simulink model "ctrl_PF_ad"  (R2023a)
settings: Solver=FixedStepAuto  StartTime=0.0  StopTime=Tf  FixedStep=0.05  RelTol=1e-3
StopFcn:
  | save('testdata')
undefined symbols (not defined in the file or in its folder): adap, Ba_0, Bb, Bv_0, Bx_0, Cp, Cp_prime, Cpv, d, dA_BP1, dA_BP2, dA_Hull, dA_PH, dA_Sail, dA_SProot, dA_X1a, dA_X1b, dA_X2a, dA_X2b, dA_X3a, dA_X3b, dA_X4a, dA_X4b, Ixx, Ixy, Ixz, Iyy, Iyz, Izz, Ky, L1, Mb, n_BP1, n_BP2, n_Hull, n_PH, n_Sail, n_SProot, n_X2a, n_X2b, n_X3a, n_X4a, n_X4b, nt_BP1, nt_BP2, nt_Hull, nt_PH, nt_Sail, nt_SProot, nt_X1a, nt_X1b, nt_X2a, nt_X2b, nt_X3a, nt_X3b, nt_X4a, nt_X4b, Seastate, Tf, Ts ... (+50)
libraries: simulink x8, sharedtransform x2, dspmathops x2
(part 2 of 5)

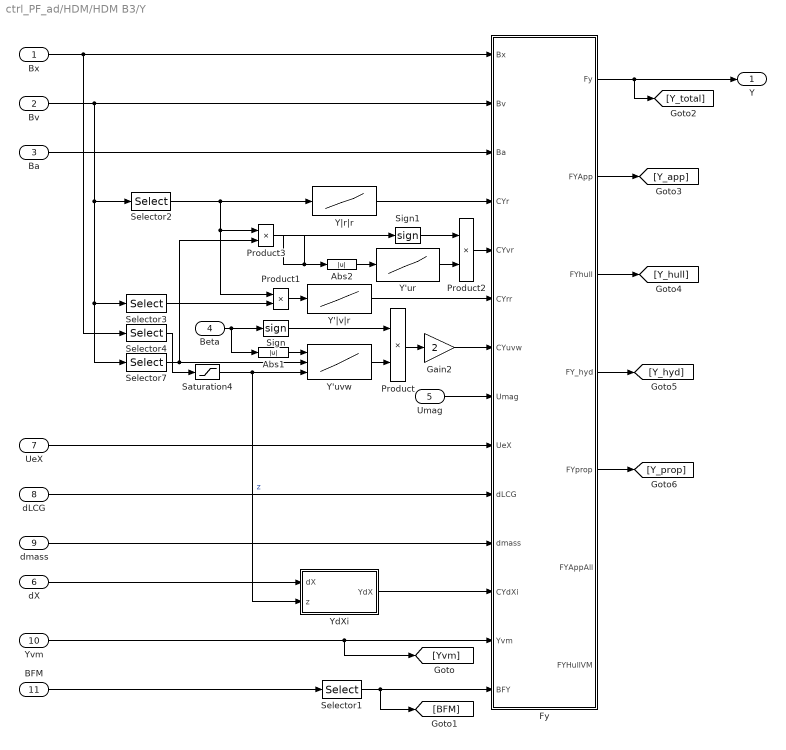
== system ctrl_PF_ad/HDM/HDM B3/Y ==
  Bx : Inport
  Bv : Inport  Port=2
  Ba : Inport  Port=3
  Beta : Inport  Port=4
  Umag : Inport  Port=5
  dX : Inport  Port=6
  UeX : Inport  Port=7
  dLCG : Inport  Port=8
  dmass : Inport  Port=9
  Yvm : Inport  Port=10
  BFM : Inport  Port=11
  Abs1 : Abs  SaturateOnIntegerOverflow=off
  Abs2 : Abs  SaturateOnIntegerOverflow=off
  Fy : MATLAB Function  TreatAsAtomicUnit=on
  Gain2 : Gain  Gain=2
  Product{,1..3} (4 alike) : Product
  Saturation4 : Saturate  UpperLimit=-13.8724  LowerLimit=-35.0624
  Selector1 : Selector  InputPortWidth=6  IndexOptions=Index vector (dialog)  Indices=2  OutputSizes=1
  Selector2 : Selector  InputPortWidth=6  IndexOptions=Index vector (dialog)  Indices=6  OutputSizes=1
  Selector3 : Selector  InputPortWidth=6  IndexOptions=Index vector (dialog)  Indices=2  OutputSizes=1
  Selector4 : Selector  InputPortWidth=6  IndexOptions=Index vector (dialog)  Indices=3  OutputSizes=1
  Selector7 : Selector  InputPortWidth=6  IndexOptions=Index vector (dialog)  Indices=1  OutputSizes=1
  Sign : Signum
  Sign1 : Signum
  Y'ur : Lookup_n-D  NumberOfTableDimensions=1  BreakpointsForDimension1=|  Table=|  InternalRulePriority=Speed  RndMeth=Simplest
      BreakpointsForDimension1=|
      | [0.03999989
      | 0.079999993
      | 0.11999963
      | 0.15999956]
      Table=|
      | [-5.2094E-04
      | -1.0594E-03
      | -1.5649E-03
      | -2.0981E-03]
  Y'uvw : Lookup_n-D  NumberOfTableDimensions=3  BreakpointsForDimension1=|  BreakpointsForDimension2=|  BreakpointsForDimension3=|  Table=|  InternalRulePriority=Speed  RndMeth=Simplest
      BreakpointsForDimension1=|
      | [0
      | 4
      | 8
      | 12]
      BreakpointsForDimension2=|
      | [-5.1444E+00
      | -3.0866E+00
      | -1.5433E+00
      | ]
      Table=|
      | reshape([0.0000000E+00
      | -5.0280621E-03
      | -9.4175348E-03
      | -1.4397458E-02
      | 0.0000000E+00
      | -5.0037454E-03
      | -9.1645405E-03
      | -1.4507402E-02
      | 0.0000000E+00
      | -4.2819107E-03
      | -9.0361786E-03
      | -1.4507235E-02
      | 0.0000000E+00
      | -4.7723270E-03
      | -9.7378407E-03
      | -1.5377541E-02
      | 0.0000000E+00
      | -4.7276301E-03
      | -9.6949815E-03
      | -1.5393721E-02
      | 0.0000000E+00
      | -4.5359209E-03
      | -9.4966039E-03
      | -1.6947859E-02
      | 0.0000000E+00
      | -5.1295007E-03
      | -1.0575377E-02
      | -1.6672924E-02
      | 0.0000000E+00
      | -4.9811404E-03
      | -1.0209461E-02
      | -1.6298327E-02
      | 0.0000000E+00
      | -4.7780219E-03
      | -1.0008968E-02
      | -1.6115181E-02
      | 0.0000000E+00
      | -5.7252015E-03
      | -1.1973447E-02
      | -1.9152812E-02
      | 0.0000000E+00
      | -5.2128737E-03
      | -1.0845978E-02
      | -1.7281669E-02
      | 0.0000000E+00
      | -4.9979037E-03
      | -1.0845685E-02
      | -1.6944141E-02],[4,3,4])
      BreakpointsForDimension3=|
      | [-35.0624 -18.3724 -15.3724 -13.8724
      | ]
      settings: InputPortMap=u0,u1,u2
  Y'|v|r : Lookup_n-D  NumberOfTableDimensions=1  BreakpointsForDimension1=|  Table=|  InternalRulePriority=Speed  RndMeth=Simplest
      BreakpointsForDimension1=|
      | [-0.0015
      | -0.0012
      | -0.0009
      | -0.0006
      | -0.0003
      | -0.0001
      | 0.0001
      | 0.0003
      | 0.0006
      | 0.0009
      | 0.0012
      | 0.0015]
      Table=|
      | [-2.9784E-01
      | -2.6725E-01
      | -2.3292E-01
      | -2.0077E-01
      | -1.1489E-01
      | -7.6673E-03
      | -7.5516E-03
      | -1.1617E-01
      | -2.0077E-01
      | -2.9128E-01
      | -3.5974E-01
      | -4.7839E-01]
  YdXi : Subsystem
  Y|r|r : Lookup_n-D  NumberOfTableDimensions=1  BreakpointsForDimension1=|  Table=|  InternalRulePriority=Speed  RndMeth=Simplest
      BreakpointsForDimension1=|
      | [-0.02
      | -0.015
      | -0.012958963
      | -0.009719222
      | -0.006479482
      | -0.003239741
      | -0.00161987
      | -0.000647948
      | 0.000647948
      | 0.00161987
      | 0.003239741
      | 0.006479482
      | 0.009719222
      | 0.012958963
      | 0.015
      | 0.02
      | ]
      Table=|
      | [3.6478E-03
      | 3.8686E-03
      | 3.4313E-03
      | 4.0790E-03
      | 3.9500E-03
      | 3.6018E-03
      | 3.6796E-03
      | 3.5502E-03
      | 3.4310E-03
      | 3.4872E-03
      | 4.2239E-03
      | 4.0934E-03
      | 3.0314E-03
      | 2.5726E-03
      | 2.9188E-03
      | 2.7740E-03
      | ]
  Y : Outport
  wires:
  Fy/5(FYprop) -> [Y_prop]
  Fy/4(FY_hyd) -> [Y_hyd]
  Fy/3(FYhull) -> [Y_hull]
  Fy/2(FYApp) -> [Y_app]
  YdXi/1(YdX) -> Fy/12(CYdXi)
  Saturation4/1 -> Y'uvw/3, YdXi/2(z)  "z"
  Selector1/1 -> Fy/14(BFY), [BFM]
  BFM/1 -> Selector1/1
  Yvm/1 -> [Yvm], Fy/13(Yvm)
  Gain2/1 -> Fy/7(CYuvw)
  Product/1 -> Gain2/1
  Abs2/1 -> Y'ur/1
  Sign1/1 -> Product2/1
  Product2/1 -> Fy/5(CYvr)
  Abs1/1 -> Y'uvw/1
  Sign/1 -> Product/1
  Y'uvw/1 -> Product/2
  Selector4/1 -> Saturation4/1
  Y'ur/1 -> Product2/2
  Y|r|r/1 -> Fy/4(CYr)
  Fy/1(Fy) -> Y/1, [Y_total]
  Y'|v|r/1 -> Fy/6(CYrr)
  Selector2/1 -> Y|r|r/1, Product3/1, Product1/1
  Product1/1 -> Y'|v|r/1
  Product3/1 -> Abs2/1, Sign1/1
  dX/1 -> YdXi/1(dX)
  dmass/1 -> Fy/11(dmass)
  dLCG/1 -> Fy/10(dLCG)
  Ba/1 -> Fy/3(Ba)
  Selector3/1 -> Product1/2
  UeX/1 -> Fy/9(UeX)
  Bx/1 -> Selector4/1, Fy/1(Bx)
  Umag/1 -> Fy/8(Umag)
  Bv/1 -> Selector7/1, Selector3/1, Selector2/1, Fy/2(Bv)
  Beta/1 -> Abs1/1, Sign/1
  Selector7/1 -> Product3/2, Y'uvw/2

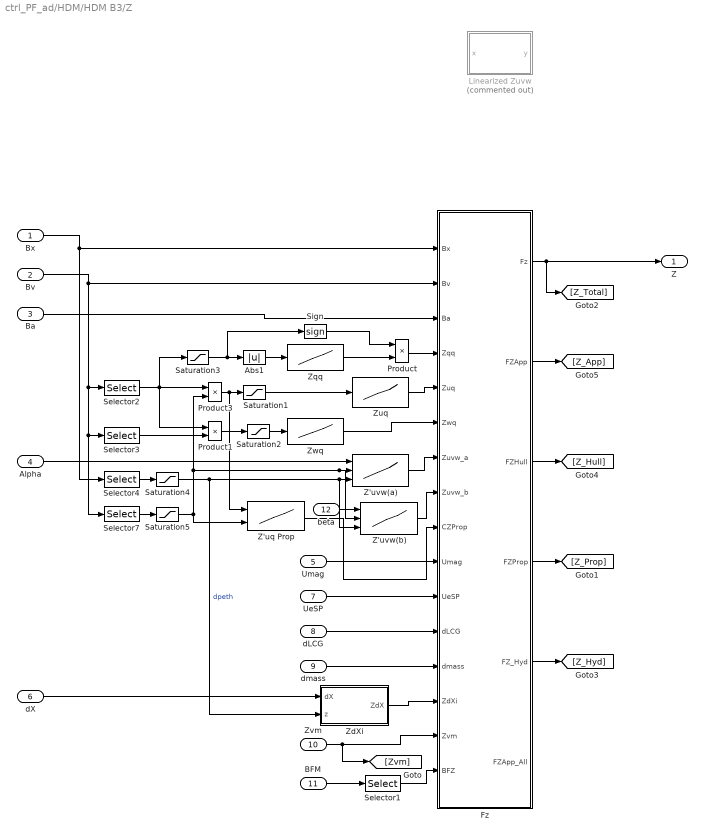
== system ctrl_PF_ad/HDM/HDM B3/Z ==
  Bx : Inport
  Bv : Inport  Port=2
  Ba : Inport  Port=3
  Alpha : Inport  Port=4
  Umag : Inport  Port=5
  dX : Inport  Port=6
  UeSP : Inport  Port=7
  dLCG : Inport  Port=8
  dmass : Inport  Port=9
  Zvm : Inport  Port=10
  BFM : Inport  Port=11
  beta : Inport  Port=12
  Abs1 : Abs  SaturateOnIntegerOverflow=off
  Fz : MATLAB Function  TreatAsAtomicUnit=on
  Linearized Zuvw : MATLAB Function  Commented=on  TreatAsAtomicUnit=on
  Product : Product
  Product1 : Product
  Product3 : Product
  Saturation1 : Saturate  UpperLimit=0.04  LowerLimit=-0.04
  Saturation2 : Saturate  UpperLimit=0.0015  LowerLimit=-0.0015
  Saturation3 : Saturate  UpperLimit=0.02  LowerLimit=-0.02
  Saturation4 : Saturate  UpperLimit=-13.8724  LowerLimit=-35.0624
  Saturation5 : Saturate  UpperLimit=-1.5433E+00  LowerLimit=-5.14444
  Selector1 : Selector  InputPortWidth=6  IndexOptions=Index vector (dialog)  Indices=3  OutputSizes=1
  Selector2 : Selector  InputPortWidth=6  IndexOptions=Index vector (dialog)  Indices=5  OutputSizes=1
  Selector3 : Selector  InputPortWidth=6  IndexOptions=Index vector (dialog)  Indices=3  OutputSizes=1
  Selector4 : Selector  InputPortWidth=6  IndexOptions=Index vector (dialog)  Indices=3  OutputSizes=1
  Selector7 : Selector  InputPortWidth=6  IndexOptions=Index vector (dialog)  Indices=1  OutputSizes=1
  Sign : Signum
  Z'uq Prop : Lookup_n-D  BreakpointsForDimension1=|  BreakpointsForDimension2=[-7.71666 -5.14444 -3.086664 -1.543332]  Table=|  InternalRulePriority=Speed  RndMeth=Simplest
      BreakpointsForDimension1=|
      | [-2.0E-01
      | -1.5E-01
      | -1.0E-01
      | -5.0E-02
      | 0.0E+00
      | 5.0E-02
      | 1.0E-01
      | 1.5E-01
      | 2.0E-01
      | ]
      Table=|
      | reshape([1.3913E-04
      | 1.0452E-04
      | 6.9900E-05
      | 3.5283E-05
      | 6.6700E-07
      | -3.3949E-05
      | -6.8566E-05
      | -1.0318E-04
      | -1.3780E-04
      | 2.8914E-04
      | 2.1702E-04
      | 1.4490E-04
      | 7.2785E-05
      | 6.6700E-07
      | -7.1451E-05
      | -1.4357E-04
      | -2.1569E-04
      | -2.8780E-04
      | 1.1606E-04
      | 8.7208E-05
      | 5.8361E-05
      | 2.9514E-05
      | 6.6700E-07
      | -2.8180E-05
      | -5.7027E-05
      | -8.5874E-05
      | -1.1472E-04
      | 1.1606E-04
      | 8.7208E-05
      | 5.8361E-05
      | 2.9514E-05
      | 6.6700E-07
      | -2.8180E-05
      | -5.7027E-05
      | -8.5874E-05
      | -1.1472E-04],[9,4])
      settings: InputPortMap=u0,u1
  Z'uvw(a) : Lookup_n-D  NumberOfTableDimensions=3  BreakpointsForDimension1=|  BreakpointsForDimension2=|  BreakpointsForDimension3=|  Table=|  InternalRulePriority=Speed  RndMeth=Simplest
      BreakpointsForDimension1=|
      | [-12
      | -8
      | -4
      | 0
      | 4
      | 8
      | 12]
      BreakpointsForDimension2=|
      | [-5.1444E+00
      | -3.0866E+00
      | -1.5433E+00
      | ]
      Table=|
      | reshape([-3.82587E-03
      | -2.42543E-03
      | -1.05453E-03
      | 1.94202E-04
      | 1.48991E-03
      | 3.04047E-03
      | 4.14104E-03
      | -3.76348E-03
      | -2.38508E-03
      | -9.82619E-04
      | 1.94202E-04
      | 1.47560E-03
      | 3.02863E-03
      | 4.06663E-03
      | -3.75964E-03
      | -2.29001E-03
      | -8.34074E-04
      | 1.94202E-04
      | 1.38956E-03
      | 2.91153E-03
      | 4.15251E-03
      | -3.11218E-03
      | -1.80502E-03
      | -4.97855E-04
      | 8.09305E-04
      | 2.11647E-03
      | 3.42363E-03
      | 4.73079E-03
      | -2.62573E-03
      | -1.48072E-03
      | -3.35708E-04
      | 8.09305E-04
      | 1.95432E-03
      | 3.09933E-03
      | 4.24434E-03
      | -2.06413E-03
      | -1.10632E-03
      | -1.48507E-04
      | 8.09305E-04
      | 1.76712E-03
      | 2.72493E-03
      | 3.68274E-03
      | -3.09997E-03
      | -1.76300E-03
      | -4.26025E-04
      | 9.10947E-04
      | 2.24792E-03
      | 3.58489E-03
      | 4.92186E-03
      | -2.49055E-03
      | -1.35672E-03
      | -2.22886E-04
      | 9.10947E-04
      | 2.04478E-03
      | 3.17861E-03
      | 4.31245E-03
      | -2.64104E-03
      | -1.45704E-03
      | -2.73048E-04
      | 9.10947E-04
      | 2.09494E-03
      | 3.27894E-03
      | 4.46293E-03
      | -0.003059752
      | -0.001711935
      | -0.000364117
      | 0.0009837
      | 0.002331518
      | 0.003679335
      | 0.005027153
      | -0.002351082
      | -0.0012256
      | -0.000100118
      | 0.0009837
      | 0.002109182
      | 0.003234664
      | 0.004360146
      | -0.001725739
      | -0.000822593
      | 8.05539E-05
      | 0.0009837
      | 0.001886847
      | 0.002789993
      | 0.00369314],[7,3,4])
      BreakpointsForDimension3=|
      | [-35.0624 -18.3724 -15.3724 -13.8724
      | ]
      settings: InputPortMap=u0,u1,u2
  Z'uvw(b) : Lookup_n-D  NumberOfTableDimensions=3  BreakpointsForDimension1=|  BreakpointsForDimension2=|  BreakpointsForDimension3=|  Table=|  InternalRulePriority=Speed  RndMeth=Simplest
      BreakpointsForDimension1=|
      | [0
      | 4
      | 8
      | 12]
      BreakpointsForDimension2=|
      | [-5.1444E+00
      | -3.0866E+00
      | -1.5433E+00
      | ]
      Table=|
      | reshape([0.0000000E+00
      | -5.9986916E-04
      | -2.7503348E-03
      | -5.0777589E-03
      | 0.0000000E+00
      | -6.0654884E-04
      | -2.4512564E-03
      | -5.2464901E-03
      | 0.0000000E+00
      | -7.6137528E-04
      | -2.4084463E-03
      | -5.2118678E-03
      | 0.0000000E+00
      | -8.2427914E-04
      | -2.5250249E-03
      | -5.3103563E-03
      | 0.0000000E+00
      | -8.1036019E-04
      | -2.5315266E-03
      | -5.5141459E-03
      | 0.0000000E+00
      | -7.9799041E-04
      | -2.5595242E-03
      | -5.2319004E-03
      | 0.0000000E+00
      | -8.6989011E-04
      | -2.5865820E-03
      | -5.6151595E-03
      | 0.0000000E+00
      | -8.4361582E-04
      | -2.6124115E-03
      | -5.7143353E-03
      | 0.0000000E+00
      | -8.2567611E-04
      | -2.6088331E-03
      | -5.6150660E-03
      | 0.0000000E+00
      | -9.1003224E-04
      | -2.7683191E-03
      | -6.0189061E-03
      | 0.0000000E+00
      | -8.4211433E-04
      | -2.5899187E-03
      | -5.7497784E-03
      | 0.0000000E+00
      | -8.2014014E-04
      | -2.4092466E-03
      | -5.6643347E-03],[4,3,4])
      BreakpointsForDimension3=|
      | [-35.0624 -18.3724 -15.3724 -13.8724
      | ]
      settings: InputPortMap=u0,u1,u2
  ZdXi : Subsystem
  Zqq : Lookup_n-D  NumberOfTableDimensions=1  BreakpointsForDimension1=|  Table=|  InternalRulePriority=Speed  RndMeth=Simplest
      BreakpointsForDimension1=|
      | [0.000127901
      | 0.000383704
      | 0.000639507
      | 0.001279013
      | 0.002558026
      | ]
      Table=|
      | [-1.5611E-03
      | -1.0379E-04
      | 3.9238E-05
      | 1.1475E-04
      | 1.3579E-04
      | ]
  Zuq : Lookup_n-D  NumberOfTableDimensions=1  BreakpointsForDimension1=|  Table=|  InternalRulePriority=Speed  RndMeth=Simplest
      BreakpointsForDimension1=|
      | [-0.04
      | -0.03
      | -0.02
      | -0.01
      | -0.005
      | -0.002
      | 0.002
      | 0.005
      | 0.01
      | 0.02
      | 0.03
      | 0.04
      | ]
      Table=|
      | [-9.8908E-03
      | -9.0784E-03
      | -8.9566E-03
      | -1.0733E-02
      | -1.4141E-02
      | -2.4189E-02
      | -6.5605E-03
      | -7.1594E-03
      | -7.6366E-03
      | -7.9008E-03
      | -6.1794E-03
      | -6.1029E-03
      | ]
  Zwq : Lookup_n-D  NumberOfTableDimensions=1  BreakpointsForDimension1=|  Table=|  InternalRulePriority=Speed  RndMeth=Simplest
      BreakpointsForDimension1=|
      | [-0.0015
      | -0.0012
      | -0.0009
      | -0.0006
      | -0.0003
      | -0.0001
      | 0.0001
      | 0.0003
      | 0.0006
      | 0.0009
      | 0.0012
      | 0.0015]
      Table=|
      | [-2.9784E-01
      | -2.6725E-01
      | -2.3292E-01
      | -2.0077E-01
      | -1.1489E-01
      | -7.6673E-03
      | -7.5516E-03
      | -1.1617E-01
      | -2.0077E-01
      | -2.9128E-01
      | -3.5974E-01
      | -4.7839E-01]
  Z : Outport
  wires:
  beta/1 -> Z'uvw(b)/1
  Z'uvw(b)/1 -> Fz/8(Zuvw_b)
  Product/1 -> Fz/4(Zqq)
  Sign/1 -> Product/1
  Abs1/1 -> Zqq/1
  Selector7/1 -> Saturation5/1
  Saturation5/1 -> Z'uq Prop/2, Z'uvw(b)/2, Z'uvw(a)/2, Product3/2
  Saturation4/1 -> ZdXi/2(z), Z'uvw(a)/3, Z'uvw(b)/3  "dpeth"
  Fz/5(FZ_Hyd) -> [Z_Hyd]
  Fz/4(FZProp) -> [Z_Prop]
  Fz/3(FZHull) -> [Z_Hull]
  Fz/2(FZApp) -> [Z_App]
  ZdXi/1(ZdX) -> Fz/14(ZdXi)
  Selector1/1 -> Fz/16(BFZ)
  BFM/1 -> Selector1/1
  Z'uvw(a)/1 -> Fz/7(Zuvw_a)
  Zqq/1 -> Product/2
  Z'uq Prop/1 -> Fz/9(CZProp)
  Zwq/1 -> Fz/6(Zwq)
  Selector2/1 -> Saturation3/1, Product1/1, Product3/1
  Alpha/1 -> Z'uvw(a)/1
  Bv/1 -> Selector7/1, Selector3/1, Selector2/1, Fz/2(Bv)
  Umag/1 -> Fz/10(Umag)
  Bx/1 -> Selector4/1, Fz/1(Bx)
  Product3/1 -> Z'uq Prop/1, Saturation1/1
  UeSP/1 -> Fz/11(UeSP)
  Selector3/1 -> Product1/2
  Product1/1 -> Saturation2/1
  dLCG/1 -> Fz/12(dLCG)
  dmass/1 -> Fz/13(dmass)
  dX/1 -> ZdXi/1(dX)
  Saturation1/1 -> Zuq/1
  Saturation2/1 -> Zwq/1
  Saturation3/1 -> Sign/1, Abs1/1
  Fz/1(Fz) -> [Z_Total], Z/1
  Zuq/1 -> Fz/5(Zuq)
  Ba/1 -> Fz/3(Ba)
  Zvm/1 -> [Zvm], Fz/15(Zvm)
  Selector4/1 -> Saturation4/1

== system ctrl_PF_ad/HDM/Integration and Coord. Transfrom/Coordinate Transform ==
  Bv : Inport
  Integrator : Integrator  InitialCondition=Bx_0
  MATLAB Function2 : MATLAB Function  TreatAsAtomicUnit=on
  X_earth : Outport  VectorParamsAs1DForOutWhenUnconnected=off
  wires:
  MATLAB Function2/1(out) -> Integrator/1
  Bv/1 -> MATLAB Function2/2(Bv)
  Integrator/1 -> X_earth/1, MATLAB Function2/1(Bx)

== system ctrl_PF_ad/HDM/Integration and Coord. Transfrom/Rigid Body Motion ==
  F_hyd : Inport
  Bx : Inport  Port=2
  Demux : Demux  Outputs=6
  Demux1 : Demux  Outputs=6
  Demux2 : Demux  Outputs=5
  Gain2 : Gain
  Integrator : Integrator  InitialCondition=Bv_0
  MATLAB Function2 : MATLAB Function  TreatAsAtomicUnit=on
  Memory1 : Memory  InitialCondition=Ba_0
  Mux1 : Mux  Inputs=6
  Mux2 : Mux  Inputs=5
  Bv : Outport  VectorParamsAs1DForOutWhenUnconnected=off
  Ba : Outport  Port=2  VectorParamsAs1DForOutWhenUnconnected=off
  wires:
  Mux1/1 -> Bv/1
  Gain2/1 -> Demux2/1
  Demux1/2 -> Mux2/1
  Demux1/4 -> Mux2/3
  Demux1/6 -> Mux2/5
  Demux1/5 -> Mux2/4
  Demux2/1 -> Mux1/2
  Demux1/1 -> Mux1/1
  Demux2/4 -> Mux1/5
  Demux2/2 -> Mux1/3
  Demux2/5 -> Mux1/6
  Mux2/1 -> Gain2/1
  Demux1/3 -> Mux2/2
  Demux2/3 -> Mux1/4
  F_hyd/1 -> Demux/1
  Demux/6 -> MATLAB Function2/6(N)
  Demux/5 -> MATLAB Function2/5(M)
  Demux/4 -> MATLAB Function2/4(K)
  Demux/3 -> MATLAB Function2/3(Z)
  Demux/2 -> MATLAB Function2/2(Y)
  Demux/1 -> MATLAB Function2/1(X)
  Memory1/1 -> Ba/1
  Integrator/1 -> Demux1/1, MATLAB Function2/8(bv)
  MATLAB Function2/1(out) -> Memory1/1, Integrator/1
  Bx/1 -> MATLAB Function2/7(bx)

== system ctrl_PF_ad/HDM/actuator saturation/  ==
  "dX " : Inport
  Constant{,3,5,7,9} (5 alike) : Constant  Value=7.11
  Constant{2,4,6,8,10} (5 alike) : Constant  Value=-7.11
  Demux3 : Demux  Outputs=5
  I-Pitch{1..5} (5 alike) : Gain
  Max Deflection{,1..4} (5 alike) : Saturate  UpperLimit=30  LowerLimit=-30
  Mux : Mux  Inputs=5
  Rate Limiter Dynamic{,1..4} (5 alike) : simulink/Discontinuities/Rate Limiter Dynamic
  Scope : Scope  NumInputPorts=5
  dX : Outport
  wires:
  Rate Limiter Dynamic3/1 -> Max Deflection3/1
  Mux/1 -> dX/1
  Constant7/1 -> Rate Limiter Dynamic3/1
  Max Deflection4/1 -> I-Pitch5/1  "dV"
  Constant8/1 -> Rate Limiter Dynamic3/3
  "dX "/1 -> Demux3/1
  Max Deflection3/1 -> I-Pitch4/1  "dV"
  Constant5/1 -> Rate Limiter Dynamic2/1
  Max Deflection1/1 -> I-Pitch1/1  "dV"
  Rate Limiter Dynamic2/1 -> Max Deflection2/1
  Constant/1 -> Rate Limiter Dynamic/1
  Rate Limiter Dynamic1/1 -> Max Deflection1/1
  Constant6/1 -> Rate Limiter Dynamic2/3
  I-Pitch4/1 -> Mux/4, Scope/4
  I-Pitch3/1 -> Mux/1, Scope/1
  Constant4/1 -> Rate Limiter Dynamic1/3
  I-Pitch1/1 -> Mux/2, Scope/2
  Max Deflection2/1 -> I-Pitch2/1  "dV"
  Rate Limiter Dynamic4/1 -> Max Deflection4/1
  I-Pitch5/1 -> Mux/5, Scope/5
  Rate Limiter Dynamic/1 -> Max Deflection/1
  Constant10/1 -> Rate Limiter Dynamic4/3
  Demux3/2 -> Rate Limiter Dynamic1/2
  Demux3/4 -> Rate Limiter Dynamic3/2
  Constant3/1 -> Rate Limiter Dynamic1/1
  Demux3/5 -> Rate Limiter Dynamic4/2
  Demux3/3 -> Rate Limiter Dynamic2/2
  Max Deflection/1 -> I-Pitch3/1  "dV"
  Demux3/1 -> Rate Limiter Dynamic/2
  Constant9/1 -> Rate Limiter Dynamic4/1
  Constant2/1 -> Rate Limiter Dynamic/3
  I-Pitch2/1 -> Mux/3, Scope/3

== system ctrl_PF_ad/HDM/actuator saturation/    ==
  "n " : Inport
  Rate Limiter Dynamic : simulink/Discontinuities/Rate Limiter Dynamic
  Rate Max : Constant  Value=14.65
  Rate Min : Constant  Value=-14.65
  Saturation6 : Saturate  UpperLimit=10  LowerLimit=0.01
  n : Outport
  wires:
  Saturation6/1 -> n/1
  Rate Max/1 -> Rate Limiter Dynamic/1
  Rate Limiter Dynamic/1 -> Saturation6/1
  Rate Min/1 -> Rate Limiter Dynamic/3
  "n "/1 -> Rate Limiter Dynamic/2

== system ctrl_PF_ad/HDM/actuator saturation/Subsystem1 ==
  dLCG : Inport
  " LCG Change Saturation" : Saturate
  Lower Rate limit : Constant  Value=-5.83e-4
  Rate Limiter Dynamic : simulink/Discontinuities/Rate Limiter Dynamic
  Upper Rate limit : Constant  Value=5.83e-4
  dLCG (m) : Outport
  wires:
  dLCG/1 -> Rate Limiter Dynamic/2
  Upper Rate limit/1 -> Rate Limiter Dynamic/1
  Lower Rate limit/1 -> Rate Limiter Dynamic/3
  Rate Limiter Dynamic/1 -> " LCG Change Saturation"/1  "dLCG (m)"
  " LCG Change Saturation"/1 -> dLCG (m)/1  "dLCG (m)"

== system ctrl_PF_ad/HDM/actuator saturation/Subsystem2 ==
  dmass : Inport
  Constant2 : Constant  Value=100
  Constant3 : Constant  Value=-100
  Max Mass Change : Saturate  UpperLimit=20000  LowerLimit=-20000
  Rate Limiter Dynamic1 : simulink/Discontinuities/Rate Limiter Dynamic
  dmass (kg) : Outport
  wires:
  Max Mass Change/1 -> dmass (kg)/1  "dmass (kg)"
  dmass/1 -> Rate Limiter Dynamic1/2
  Constant2/1 -> Rate Limiter Dynamic1/1
  Rate Limiter Dynamic1/1 -> Max Mass Change/1  "dmass (kg)"
  Constant3/1 -> Rate Limiter Dynamic1/3

== system ctrl_PF_ad/HDM/HDM B3/K/KdXi ==
  dX : Inport
  UeX : Inport  Port=2
  z : Inport  Port=3
  KdX1 : Lookup_n-D  NumberOfTableDimensions=3  BreakpointsForDimension1=[-10 0 10]  BreakpointsForDimension2=|  BreakpointsForDimension3=[-5.14444 -3.08666664 -1.54332]  Table=|  InternalRulePriority=Speed  RndMeth=Simplest
      BreakpointsForDimension2=|
      | [-36.4062987
      | -18.4062987
      | -15.4062987
      | -13.9062987]
      Table=|
      | reshape([-3.9047E-05
      | 4.5684E-07
      | 3.9769E-05
      | -3.8309E-05
      | 1.2643E-06
      | 4.0809E-05
      | -3.0256E-05
      | 1.2643E-06
      | 4.8387E-05
      | -3.7558E-05
      | 2.1545E-06
      | 4.2083E-05
      | -3.9057E-05
      | 3.6064E-07
      | 3.9562E-05
      | -3.8473E-05
      | 1.0476E-06
      | 4.0437E-05
      | -3.0256E-05
      | 1.4418E-06
      | 4.8387E-05
      | -3.7906E-05
      | 1.7415E-06
      | 4.1434E-05
      | -3.8945E-05
      | 2.8249E-07
      | 3.9429E-05
      | -3.8396E-05
      | 9.1134E-07
      | 4.0237E-05
      | -3.8190E-05
      | 9.1134E-07
      | 4.0733E-05
      | -3.7932E-05
      | 1.5343E-06
      | 4.1020E-05
      | ],[3,4,3])
      settings: InputPortMap=u0,u1,u2
  KdX2 : Lookup_n-D  NumberOfTableDimensions=3  BreakpointsForDimension1=[-10 0 10]  BreakpointsForDimension2=|  BreakpointsForDimension3=[-5.14444 -3.08666664 -1.54332]  Table=|  InternalRulePriority=Speed  RndMeth=Simplest
      BreakpointsForDimension2=|
      | [-36.4062987
      | -18.4062987
      | -15.4062987
      | -13.9062987]
      Table=|
      | reshape([-3.5775E-05
      | -2.4080E-07
      | 3.3150E-05
      | -3.4263E-05
      | 1.2268E-06
      | 3.5342E-05
      | -2.3577E-05
      | 1.2268E-06
      | 4.6338E-05
      | -3.2368E-05
      | 3.5682E-06
      | 3.9469E-05
      | -3.5785E-05
      | -3.3131E-07
      | 3.3067E-05
      | -3.4544E-05
      | 8.9010E-07
      | 3.4889E-05
      | -2.3577E-05
      | 1.7076E-06
      | 4.6338E-05
      | -3.3141E-05
      | 2.4187E-06
      | 3.7389E-05
      | -3.5809E-05
      | -5.7189E-07
      | 3.3046E-05
      | -3.4706E-05
      | 4.2723E-07
      | 3.4588E-05
      | -3.4017E-05
      | 4.2723E-07
      | 3.5657E-05
      | -3.3562E-05
      | 1.6134E-06
      | 3.6605E-05
      | ],[3,4,3])
      settings: InputPortMap=u0,u1,u2
  KdX3 : Lookup_n-D  NumberOfTableDimensions=3  BreakpointsForDimension1=[-10 0 10]  BreakpointsForDimension2=|  BreakpointsForDimension3=[-5.14444 -3.08666664 -1.54332]  Table=|  InternalRulePriority=Speed  RndMeth=Simplest
      BreakpointsForDimension2=|
      | [-36.4062987
      | -18.4062987
      | -15.4062987
      | -13.9062987]
      Table=|
      | reshape([-4.3139E-05
      | 1.7292E-07
      | 4.5001E-05
      | -4.4081E-05
      | -1.2796E-06
      | 4.2448E-05
      | -4.9749E-05
      | -1.2796E-06
      | 2.6691E-05
      | -4.5613E-05
      | -3.5861E-06
      | 3.8362E-05
      | -4.2707E-05
      | 2.7384E-07
      | 4.4575E-05
      | -4.3360E-05
      | -9.3523E-07
      | 4.2465E-05
      | -4.9749E-05
      | -1.7362E-06
      | 2.6691E-05
      | -4.4279E-05
      | -2.4363E-06
      | 3.9821E-05
      | -4.1687E-05
      | 5.3371E-07
      | 4.3082E-05
      | -4.2289E-05
      | -4.5361E-07
      | 4.1207E-05
      | -4.2616E-05
      | -4.5361E-07
      | 4.0204E-05
      | -4.2521E-05
      | -1.6159E-06
      | 3.9463E-05
      | ],[3,4,3])
      settings: InputPortMap=u0,u1,u2
  KdX4 : Lookup_n-D  NumberOfTableDimensions=3  BreakpointsForDimension1=[-10 0 10]  BreakpointsForDimension2=|  BreakpointsForDimension3=[-5.14444 -3.08666664 -1.54332]  Table=|  InternalRulePriority=Speed  RndMeth=Simplest
      BreakpointsForDimension2=|
      | [-36.4062987
      | -18.4062987
      | -15.4062987
      | -13.9062987]
      Table=|
      | reshape([-4.0969E-05
      | -4.5313E-07
      | 4.0019E-05
      | -4.1787E-05
      | -1.2714E-06
      | 3.9006E-05
      | -4.8908E-05
      | -1.2714E-06
      | 3.0663E-05
      | -4.2681E-05
      | -2.1920E-06
      | 3.7920E-05
      | -4.0777E-05
      | -3.6185E-07
      | 4.0047E-05
      | -4.1470E-05
      | -1.0577E-06
      | 3.9147E-05
      | -4.8908E-05
      | -1.4679E-06
      | 3.0663E-05
      | -4.2187E-05
      | -1.7779E-06
      | 3.8312E-05
      | -4.0496E-05
      | -2.8854E-07
      | 4.0049E-05
      | -4.1082E-05
      | -9.2714E-07
      | 3.9223E-05
      | -4.1472E-05
      | -9.2714E-07
      | 3.8784E-05
      | -4.1733E-05
      | -1.5768E-06
      | 3.8383E-05
      | ],[3,4,3])
      settings: InputPortMap=u0,u1,u2
  Mux : Mux
  Selector1 : Selector  InputPortWidth=5  IndexOptions=Index vector (dialog)  Indices=2  OutputSizes=1
  Selector2 : Selector  InputPortWidth=5  IndexOptions=Index vector (dialog)  Indices=3  OutputSizes=1
  Selector3 : Selector  InputPortWidth=5  IndexOptions=Index vector (dialog)  Indices=4  OutputSizes=1
  Selector4 : Selector  InputPortWidth=5  IndexOptions=Index vector (dialog)  Indices=1  OutputSizes=1
  Selector5 : Selector  InputPortWidth=5  IndexOptions=Index vector (dialog)  Indices=2  OutputSizes=1
  Selector6 : Selector  InputPortWidth=5  IndexOptions=Index vector (dialog)  Indices=3  OutputSizes=1
  Selector7 : Selector  InputPortWidth=5  IndexOptions=Index vector (dialog)  Indices=1  OutputSizes=1
  Selector8 : Selector  InputPortWidth=5  IndexOptions=Index vector (dialog)  Indices=4  OutputSizes=1
  KdXi : Outport
  wires:
  Selector5/1 -> KdX2/3
  Selector6/1 -> KdX3/3
  Selector8/1 -> KdX4/3
  Selector4/1 -> KdX1/3
  UeX/1 -> Selector4/1, Selector5/1, Selector8/1, Selector6/1
  Selector3/1 -> KdX4/1
  Selector2/1 -> KdX3/1
  Selector1/1 -> KdX2/1
  KdX4/1 -> Mux/4
  KdX3/1 -> Mux/3
  KdX2/1 -> Mux/2
  KdX1/1 -> Mux/1
  z/1 -> KdX1/2, KdX2/2, KdX3/2, KdX4/2
  Mux/1 -> KdXi/1
  Selector7/1 -> KdX1/1
  dX/1 -> Selector7/1, Selector2/1, Selector3/1, Selector1/1

== system ctrl_PF_ad/HDM/HDM B3/M/Mdxi ==
  dX : Inport
  z : Inport  Port=2
  Demux6 : Demux  Outputs=5
  Gain{,1..4} (5 alike) : Gain
  Mux : Mux  Inputs=5
  ZudX1 q+1 : Lookup_n-D  BreakpointsForDimension1=[-30 -20 -10 0 10 20 30]  BreakpointsForDimension2=[-35.0624 -15.3724 -13.8724]  BreakpointsForDimension3=[-5.14444 -3.08666664 -1.54332]  Table=|  InternalRulePriority=Speed  RndMeth=Simplest
      | reshape([0.000594819
      | 0.000394915
      | 0.000195011
      | -4.89222E-06
      | -0.000204796
      | -0.0004047
      | -0.000604603
      | 0.000596203
      | 0.000392018
      | 0.000187833
      | -1.6352E-05
      | -0.000220537
      | -0.000424722
      | -0.000628907
      | 0.000582351
      | 0.000381446
      | 0.000180542
      | -2.03625E-05
      | -0.000221267
      | -0.000422171
      | -0.000623076
      | ],[7,3])
      settings: InputPortMap=u0,u1
  ZudX1 q+2 : Lookup_n-D  BreakpointsForDimension1=[-30 -20 -10 0 10 20 30]  BreakpointsForDimension2=[-35.0624 -15.3724 -13.8724]  BreakpointsForDimension3=[-5.14444 -3.08666664 -1.54332]  Table=|  InternalRulePriority=Speed  RndMeth=Simplest
      | reshape([0.000583784
      | 0.000394316
      | 0.000204847
      | 1.53782E-05
      | -0.000174091
      | -0.000363559
      | -0.000553028
      | 0.00056228
      | 0.000374724
      | 0.000187169
      | -3.86644E-07
      | -0.000187942
      | -0.000375498
      | -0.000563053
      | 0.000546298
      | 0.000362052
      | 0.000177806
      | -6.43933E-06
      | -0.000190685
      | -0.000374931
      | -0.000559176],[7,3])
      settings: InputPortMap=u0,u1
  ZudX1 q+3 : Lookup_n-D  BreakpointsForDimension1=[-30 -20 -10 0 10 20 30]  BreakpointsForDimension2=[-35.0624 -15.3724 -13.8724]  BreakpointsForDimension3=[-5.14444 -3.08666664 -1.54332]  Table=|  InternalRulePriority=Speed  RndMeth=Simplest
      | reshape([-0.000586989
      | -0.000395541
      | -0.000204094
      | -1.26467E-05
      | 0.000178801
      | 0.000370248
      | 0.000561695
      | -0.000568868
      | -0.000379268
      | -0.000189669
      | -6.86388E-08
      | 0.000189531
      | 0.000379131
      | 0.000568731
      | -0.000565299
      | -0.000378949
      | -0.000192598
      | -6.24776E-06
      | 0.000180103
      | 0.000366453
      | 0.000552804],[7,3])
      settings: InputPortMap=u0,u1
  ZudX1 q+4 : Lookup_n-D  BreakpointsForDimension1=[-30 -20 -10 0 10 20 30]  BreakpointsForDimension2=[-35.0624 -15.3724 -13.8724]  BreakpointsForDimension3=[-5.14444 -3.08666664 -1.54332]  Table=|  InternalRulePriority=Speed  RndMeth=Simplest
      | reshape([-0.000638396
      | -0.000426715
      | -0.000215035
      | -3.35454E-06
      | 0.000208326
      | 0.000420006
      | 0.000631687
      | -0.000598951
      | -0.000393944
      | -0.000188937
      | 1.60698E-05
      | 0.000221077
      | 0.000426084
      | 0.000631091
      | -0.000622514
      | -0.000421726
      | -0.000220939
      | -2.01522E-05
      | 0.000180635
      | 0.000381422
      | 0.000582209],[7,3])
      settings: InputPortMap=u0,u1
  ZudX1 q+5 : Lookup_n-D  BreakpointsForDimension1=[-30 -20 -10 0 10 20 30]  BreakpointsForDimension2=[-35.0624 -15.3724 -13.8724]  BreakpointsForDimension3=[-35.0624 -15.3724 -13.8724]  Table=|  InternalRulePriority=Speed  RndMeth=Simplest
      | reshape([-0.000461714
      | -0.000296336
      | -0.000130959
      | 3.44194E-05
      | 0.000199797
      | 0.000365175
      | 0.000530553
      | -0.000503641
      | -0.000327652
      | -0.000151663
      | 2.43257E-05
      | 0.000200315
      | 0.000376303
      | 0.000552292
      | -0.000536558
      | -0.000356664
      | -0.00017677
      | 3.1235E-06
      | 0.000183017
      | 0.000362911
      | 0.000542805],[7,3])
      settings: InputPortMap=u0,u1
  MdX : Outport
  wires:
  Gain4/1 -> Mux/5
  Gain1/1 -> Mux/4
  Gain2/1 -> Mux/3
  Gain3/1 -> Mux/2
  Gain/1 -> Mux/1
  dX/1 -> Demux6/1
  Demux6/1 -> ZudX1 q+1/1
  Mux/1 -> MdX/1
  z/1 -> ZudX1 q+1/2, ZudX1 q+2/2, ZudX1 q+3/2, ZudX1 q+4/2, ZudX1 q+5/2
  ZudX1 q+5/1 -> Gain4/1
  ZudX1 q+1/1 -> Gain/1
  ZudX1 q+2/1 -> Gain3/1
  ZudX1 q+3/1 -> Gain2/1
  ZudX1 q+4/1 -> Gain1/1
  Demux6/2 -> ZudX1 q+2/1
  Demux6/3 -> ZudX1 q+3/1
  Demux6/4 -> ZudX1 q+4/1
  Demux6/5 -> ZudX1 q+5/1

== system ctrl_PF_ad/HDM/HDM B3/N/NdXi ==
  dX : Inport
  z : Inport  Port=2
  Mux : Mux
  NdX1 : Lookup_n-D  BreakpointsForDimension1=[-10 0 10]  BreakpointsForDimension2=|  BreakpointsForDimension3=[-5.14444 -3.08666664 -1.54332]  Table=|  InternalRulePriority=Speed  RndMeth=Simplest
      BreakpointsForDimension2=|
      | [-36.4062987
      | -18.4062987
      | -15.4062987
      | -13.9062987]
      Table=|
      | reshape([-8.13475E-05
      | -3.25752E-06
      | 6.9363E-05
      | -8.00129E-05
      | -1.7093E-06
      | 7.14001E-05
      | -6.46417E-05
      | -1.7093E-06
      | 8.57128E-05
      | -7.85432E-05
      | -1.19372E-08
      | 7.37459E-05],[3,4])
      settings: InputPortMap=u0,u1
  NdX2 : Lookup_n-D  BreakpointsForDimension1=[-10 0 10]  BreakpointsForDimension2=|  BreakpointsForDimension3=[-5.14444 -3.08666664 -1.54332]  Table=|  InternalRulePriority=Speed  RndMeth=Simplest
      BreakpointsForDimension2=|
      | [-36.4062987
      | -18.4062987
      | -15.4062987
      | -13.9062987]
      Table=|
      | reshape([6.2278E-05
      | -3.5277E-06
      | -7.1028E-05
      | 5.9473E-05
      | -6.2352E-06
      | -7.5067E-05
      | 3.9525E-05
      | -6.2352E-06
      | -9.4282E-05
      | 5.5892E-05
      | -1.0640E-05
      | -8.2654E-05],[3,4])
      settings: InputPortMap=u0,u1
  NdX3 : Lookup_n-D  BreakpointsForDimension1=[-10 0 10]  BreakpointsForDimension2=|  BreakpointsForDimension3=[-5.14444 -3.08666664 -1.54332]  Table=|  InternalRulePriority=Speed  RndMeth=Simplest
      BreakpointsForDimension2=|
      | [-36.4062987
      | -18.4062987
      | -15.4062987
      | -13.9062987]
      Table=|
      | reshape([8.96891E-05
      | 3.65995E-06
      | -8.07998E-05
      | 9.13096E-05
      | 6.34009E-06
      | -7.59117E-05
      | 0.000100356
      | 6.34009E-06
      | -4.56822E-05
      | 9.40576E-05
      | 1.06795E-05
      | -6.79415E-05],[3,4])
      settings: InputPortMap=u0,u1
  NdX4 : Lookup_n-D  BreakpointsForDimension1=[-10 0 10]  BreakpointsForDimension2=|  BreakpointsForDimension3=[-5.14444 -3.08666664 -1.54332]  Table=|  InternalRulePriority=Speed  RndMeth=Simplest
      BreakpointsForDimension2=|
      | [-36.4062987
      | -18.4062987
      | -15.4062987
      | -13.9062987]
      Table=|
      | reshape([-7.16232E-05
      | 3.25314E-06
      | 8.32589E-05
      | -7.3213E-05
      | 1.68586E-06
      | 8.13825E-05
      | -8.66615E-05
      | 1.68586E-06
      | 6.54218E-05
      | -7.48528E-05
      | -6.7812E-08
      | 7.92559E-05],[3,4])
      settings: InputPortMap=u0,u1
  Selector1 : Selector  InputPortWidth=5  IndexOptions=Index vector (dialog)  Indices=2  OutputSizes=1
  Selector2 : Selector  InputPortWidth=5  IndexOptions=Index vector (dialog)  Indices=3  OutputSizes=1
  Selector3 : Selector  InputPortWidth=5  IndexOptions=Index vector (dialog)  Indices=4  OutputSizes=1
  Selector7 : Selector  InputPortWidth=5  IndexOptions=Index vector (dialog)  Indices=1  OutputSizes=1
  NdXi : Outport
  wires:
  Selector3/1 -> NdX4/1
  Selector2/1 -> NdX3/1
  Selector1/1 -> NdX2/1
  NdX4/1 -> Mux/4
  NdX3/1 -> Mux/3
  NdX2/1 -> Mux/2
  NdX1/1 -> Mux/1
  z/1 -> NdX1/2, NdX2/2, NdX3/2, NdX4/2
  Mux/1 -> NdXi/1
  Selector7/1 -> NdX1/1
  dX/1 -> Selector7/1, Selector1/1, Selector2/1, Selector3/1

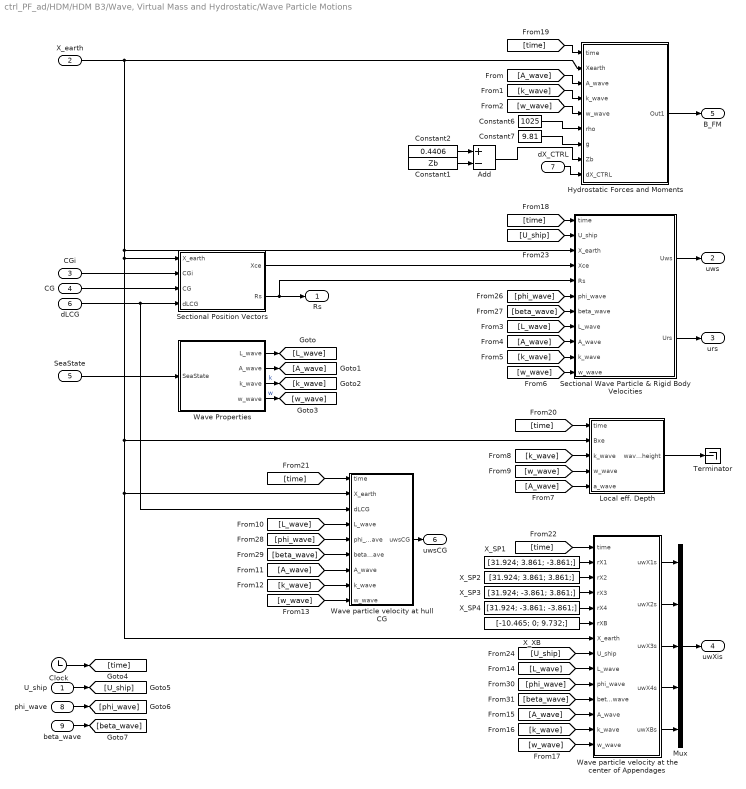
== system ctrl_PF_ad/HDM/HDM B3/Wave, Virtual Mass and Hydrostatic/Wave Particle Motions ==
  U_ship : Inport
  X_earth : Inport  Port=2
  CGi : Inport  Port=3
  CG : Inport  Port=4
  SeaState : Inport  Port=5
  dLCG : Inport  Port=6
  dX_CTRL : Inport  Port=7
  phi_wave : Inport  Port=8
  beta_wave : Inport  Port=9
  Add : Sum  Inputs=+-
  Clock : Clock
  Constant1 : Constant  Value=Zb
  Constant2 : Constant  Value=0.4406
  Constant6 : Constant  Value=1025
  Constant7 : Constant  Value=9.81
  Hydrostatic Forces and Moments : Subsystem
  Local eff. Depth : MATLAB Function  TreatAsAtomicUnit=on
  Mux : Mux  Inputs=5
  Sectional Position Vectors : MATLAB Function  TreatAsAtomicUnit=on
  Sectional Wave Particle & Rigid Body Velocities : MATLAB Function  TreatAsAtomicUnit=on
  Terminator : Terminator
  Wave Properties : MATLAB Function  TreatAsAtomicUnit=on
  Wave particle velocity at hull CG : MATLAB Function  TreatAsAtomicUnit=on
  Wave particle velocity at the center of Appendages : MATLAB Function  TreatAsAtomicUnit=on
  X_SP1 : Constant  Value=[31.924; 3.861; -3.861;]
  X_SP2 : Constant  Value=[31.924; 3.861; 3.861;]
  X_SP3 : Constant  Value=[31.924; -3.861; 3.861;]
  X_SP4 : Constant  Value=[31.924; -3.861; -3.861;]
  X_XB : Constant  Value=[-10.465; 0; 9.732;]
  Rs : Outport
  uws : Outport  Port=2
  urs : Outport  Port=3
  uwXis : Outport  Port=4
  B_FM : Outport  Port=5
  uwsCG : Outport  Port=6
  wires:
  [beta_wave] -> Wave particle velocity at the center of Appendages/11(beta_wave)
  [phi_wave] -> Wave particle velocity at the center of Appendages/10(phi_wave)
  [beta_wave] -> Wave particle velocity at hull CG/6(beta_wave)
  [phi_wave] -> Wave particle velocity at hull CG/5(phi_wave)
  [beta_wave] -> Sectional Wave Particle & Rigid Body Velocities/7(beta_wave)
  [phi_wave] -> Sectional Wave Particle & Rigid Body Velocities/6(phi_wave)
  beta_wave/1 -> [beta_wave]
  phi_wave/1 -> [phi_wave]
  [U_ship] -> Wave particle velocity at the center of Appendages/8(U_ship)
  [U_ship] -> Sectional Wave Particle & Rigid Body Velocities/2(U_ship)
  U_ship/1 -> [U_ship]
  [time] -> Wave particle velocity at the center of Appendages/1(time)
  [time] -> Wave particle velocity at hull CG/1(time)
  [time] -> Local eff. Depth/1(time)
  [time] -> Hydrostatic Forces and Moments/1(time)
  [time] -> Sectional Wave Particle & Rigid Body Velocities/1(time)
  Clock/1 -> [time]
  [w_wave] -> Wave particle velocity at the center of Appendages/14(w_wave)
  [k_wave] -> Wave particle velocity at the center of Appendages/13(k_wave)
  [A_wave] -> Wave particle velocity at the center of Appendages/12(A_wave)
  [L_wave] -> Wave particle velocity at the center of Appendages/9(L_wave)
  [w_wave] -> Wave particle velocity at hull CG/9(w_wave)
  [k_wave] -> Wave particle velocity at hull CG/8(k_wave)
  [A_wave] -> Wave particle velocity at hull CG/7(A_wave)
  [L_wave] -> Wave particle velocity at hull CG/4(L_wave)
  [w_wave] -> Local eff. Depth/4(w_wave)
  [A_wave] -> Local eff. Depth/5(a_wave)
  [k_wave] -> Local eff. Depth/3(k_wave)
  [w_wave] -> Sectional Wave Particle & Rigid Body Velocities/11(w_wave)
  [k_wave] -> Sectional Wave Particle & Rigid Body Velocities/10(k_wave)
  [A_wave] -> Sectional Wave Particle & Rigid Body Velocities/9(A_wave)
  [L_wave] -> Sectional Wave Particle & Rigid Body Velocities/8(L_wave)
  [w_wave] -> Hydrostatic Forces and Moments/5(w_wave)
  [k_wave] -> Hydrostatic Forces and Moments/4(k_wave)
  [A_wave] -> Hydrostatic Forces and Moments/3(A_wave)
  Wave Properties/4(w_wave) -> [w_wave]  "w"
  Wave Properties/3(k_wave) -> [k_wave]  "k"
  Wave Properties/2(A_wave) -> [A_wave]
  Wave Properties/1(L_wave) -> [L_wave]
  dX_CTRL/1 -> Hydrostatic Forces and Moments/9(dX_CTRL)
  Constant1/1 -> Add/2
  Constant2/1 -> Add/1
  Add/1 -> Hydrostatic Forces and Moments/8(Zb)
  Constant7/1 -> Hydrostatic Forces and Moments/7(g)
  Constant6/1 -> Hydrostatic Forces and Moments/6(rho)
  Hydrostatic Forces and Moments/1(Out1) -> B_FM/1
  Wave particle velocity at hull CG/1(uwsCG) -> uwsCG/1
  Mux/1 -> uwXis/1
  Wave particle velocity at the center of Appendages/5(uwXBs) -> Mux/5
  Wave particle velocity at the center of Appendages/4(uwX4s) -> Mux/4
  Wave particle velocity at the center of Appendages/3(uwX3s) -> Mux/3
  Wave particle velocity at the center of Appendages/2(uwX2s) -> Mux/2
  Wave particle velocity at the center of Appendages/1(uwX1s) -> Mux/1
  X_SP1/1 -> Wave particle velocity at the center of Appendages/2(rX1)
  X_SP2/1 -> Wave particle velocity at the center of Appendages/3(rX2)
  X_SP3/1 -> Wave particle velocity at the center of Appendages/4(rX3)
  X_SP4/1 -> Wave particle velocity at the center of Appendages/5(rX4)
  X_XB/1 -> Wave particle velocity at the center of Appendages/6(rXB)
  Local eff. Depth/1(wave_height) -> Terminator/1
  dLCG/1 -> Sectional Position Vectors/4(dLCG), Wave particle velocity at hull CG/3(dLCG)
  Sectional Wave Particle & Rigid Body Velocities/1(Uws) -> uws/1
  Sectional Wave Particle & Rigid Body Velocities/2(Urs) -> urs/1
  CG/1 -> Sectional Position Vectors/3(CG)
  CGi/1 -> Sectional Position Vectors/2(CGi)
  X_earth/1 -> Hydrostatic Forces and Moments/2(Xearth), Sectional Wave Particle & Rigid Body Velocities/3(X_earth), Sectional Position Vectors/1(X_earth), Local eff. Depth/2(Bxe), Wave particle velocity at the center of Appendages/7(X_earth), Wave particle velocity at hull CG/2(X_earth)
  Sectional Position Vectors/1(Xce) -> Sectional Wave Particle & Rigid Body Velocities/4(Xce)
  SeaState/1 -> Wave Properties/1(SeaState)
  Sectional Position Vectors/2(Rs) -> Sectional Wave Particle & Rigid Body Velocities/5(Rs), Rs/1

== system ctrl_PF_ad/HDM/HDM B3/X/X'dXi ==
  UeX : Inport
  dXeff : Inport  Port=2
  Gain : Gain  Gain=-1
  Gain{4..7} (4 alike) : Gain
  Mux : Mux  Inputs=5
  Saturation6 : Saturate  UpperLimit=-1.543332  LowerLimit=-5.14444
  Selector10 : Selector  InputPortWidth=5  IndexOptions=Index vector (dialog)  Indices=4  OutputSizes=1
  Selector11 : Selector  InputPortWidth=5  IndexOptions=Index vector (dialog)  Indices=4  OutputSizes=1
  Selector12 : Selector  InputPortWidth=5  IndexOptions=Index vector (dialog)  Indices=5  OutputSizes=1
  Selector2 : Selector  InputPortWidth=5  IndexOptions=Index vector (dialog)  Indices=5  OutputSizes=1
  Selector4 : Selector  InputPortWidth=5  IndexOptions=Index vector (dialog)  Indices=1  OutputSizes=1
  Selector5 : Selector  InputPortWidth=5  IndexOptions=Index vector (dialog)  Indices=1  OutputSizes=1
  Selector6 : Selector  InputPortWidth=5  IndexOptions=Index vector (dialog)  Indices=2  OutputSizes=1
  Selector7 : Selector  InputPortWidth=5  IndexOptions=Index vector (dialog)  Indices=2  OutputSizes=1
  Selector8 : Selector  InputPortWidth=5  IndexOptions=Index vector (dialog)  Indices=3  OutputSizes=1
  Selector9 : Selector  InputPortWidth=5  IndexOptions=Index vector (dialog)  Indices=3  OutputSizes=1
  XudX1 : Lookup_n-D  BreakpointsForDimension1=[-30 -20 -10 0 10 20 30]  BreakpointsForDimension2=|  Table=|  InternalRulePriority=Speed  RndMeth=Simplest
      BreakpointsForDimension2=|
      | [-7.716666
      | -5.144444
      | -3.0866664
      | -1.5433332
      | ]
      Table=|
      | reshape([3.2151E-04
      | 1.4055E-04
      | 2.3723E-05
      | -2.9685E-05
      | 2.3777E-05
      | 1.3375E-04
      | 3.3722E-04
      | 1.6076E-04
      | 7.0275E-05
      | 1.1862E-05
      | -1.4843E-05
      | 1.1889E-05
      | 6.6875E-05
      | 1.6861E-04
      | 1.6698E-04
      | 6.8790E-05
      | 1.2322E-05
      | -1.4312E-05
      | 1.2274E-05
      | 6.7265E-05
      | 1.7083E-04
      | 3.4224E-04
      | 1.3333E-04
      | 2.5937E-05
      | -6.5668E-05
      | 2.5937E-05
      | 1.3102E-04
      | 3.4214E-04
      | ],[7,4])
      settings: InputPortMap=u0,u1
  XudX2 : Lookup_n-D  BreakpointsForDimension1=[-30 -20 -10 0 10 20 30]  BreakpointsForDimension2=|  Table=|  InternalRulePriority=Speed  RndMeth=Simplest
      BreakpointsForDimension2=|
      | [-7.716666
      | -5.144444
      | -3.0866664
      | -1.5433332
      | ]
      Table=|
      | reshape([2.9233E-04
      | 1.3189E-04
      | 2.3224E-05
      | -2.9022E-05
      | 1.9675E-05
      | 1.4726E-04
      | 3.7676E-04
      | 1.4617E-04
      | 6.5945E-05
      | 1.1612E-05
      | -1.4511E-05
      | 9.8375E-06
      | 7.3630E-05
      | 1.8838E-04
      | 1.7319E-04
      | 6.7285E-05
      | 1.2060E-05
      | -2.5958E-05
      | 1.0337E-05
      | 7.6660E-05
      | 1.8963E-04
      | 3.4748E-04
      | 1.3335E-04
      | 2.2395E-05
      | -2.6403E-05
      | 2.2395E-05
      | 1.5181E-04
      | 3.8598E-04
      | ],[7,4])
      settings: InputPortMap=u0,u1
  XudX3 : Lookup_n-D  BreakpointsForDimension1=[-30 -20 -10 0 10 20 30]  BreakpointsForDimension2=|  Table=|  InternalRulePriority=Speed  RndMeth=Simplest
      BreakpointsForDimension2=|
      | [-7.716666
      | -5.144444
      | -3.0866664
      | -1.5433332
      | ]
      Table=|
      | reshape([3.5642E-04
      | 1.5674E-04
      | 2.5449E-05
      | -2.9060E-05
      | 2.6726E-05
      | 1.6225E-04
      | 3.1115E-04
      | 1.7821E-04
      | 7.8370E-05
      | 1.2725E-05
      | -1.4530E-05
      | 1.3363E-05
      | 8.1125E-05
      | 1.5558E-04
      | 1.9053E-04
      | 8.0600E-05
      | 1.2911E-05
      | -1.3998E-05
      | 1.3672E-05
      | 7.4645E-05
      | 1.6290E-04
      | 3.8447E-04
      | 1.4526E-04
      | 2.7824E-05
      | -2.6434E-05
      | 2.7824E-05
      | 1.5039E-04
      | 3.2499E-04
      | ],[7,4])
      settings: InputPortMap=u0,u1
  XudX4 : Lookup_n-D  BreakpointsForDimension1=[-30 -20 -10 0 10 20 30]  BreakpointsForDimension2=|  Table=|  InternalRulePriority=Speed  RndMeth=Simplest
      BreakpointsForDimension2=|
      | [-7.716666
      | -5.144444
      | -3.0866664
      | -1.5433332
      | ]
      Table=|
      | reshape([3.4525E-04
      | 1.3840E-04
      | 2.4668E-05
      | -2.9702E-05
      | 2.4205E-05
      | 1.2737E-04
      | 3.2790E-04
      | 1.7263E-04
      | 6.9200E-05
      | 1.2334E-05
      | -1.4851E-05
      | 1.2103E-05
      | 6.3685E-05
      | 1.6395E-04
      | 1.7298E-04
      | 6.9435E-05
      | 1.2696E-05
      | -1.4315E-05
      | 1.2608E-05
      | 6.9175E-05
      | 1.6779E-04
      | 3.3803E-04
      | 1.5513E-04
      | 2.6677E-05
      | -2.7052E-05
      | 2.6677E-05
      | 1.3644E-04
      | 3.3780E-04
      | ],[7,4])
      settings: InputPortMap=u0,u1
  XudXB : Lookup_n-D  BreakpointsForDimension1=[-30 -20 -10 0 10 20 30]  BreakpointsForDimension2=[-5.14444 -3.08666664 -1.54332]  Table=|  InternalRulePriority=Speed  RndMeth=Simplest
      | reshape([6.9060E-04
      | 3.9256E-04
      | 1.5651E-04
      | 0.0000E+00
      | 1.1449E-04
      | 4.2412E-04
      | 5.7370E-04
      | 6.4542E-04
      | 3.9138E-04
      | 1.5593E-04
      | 0.0000E+00
      | 1.1381E-04
      | 4.1205E-04
      | 5.6813E-04
      | 6.5675E-04
      | 3.9410E-04
      | 1.1271E-04
      | 0.0000E+00
      | 1.1271E-04
      | 4.2649E-04
      | 5.7604E-04
      | ],[7,3])
      settings: InputPortMap=u0,u1
  Out1 : Outport
  wires:
  Saturation6/1 -> Selector5/1, Selector7/1, Selector9/1, Selector12/1, Selector11/1
  Gain/1 -> Saturation6/1
  XudXB/1 -> Mux/5
  Gain7/1 -> Mux/4
  Gain5/1 -> Mux/3
  Gain6/1 -> Mux/2
  Gain4/1 -> Mux/1
  Selector12/1 -> XudXB/2
  Selector10/1 -> XudX4/1
  Selector11/1 -> XudX4/2
  UeX/1 -> Gain/1
  Selector9/1 -> XudX3/2
  Selector8/1 -> XudX3/1
  Selector7/1 -> XudX2/2
  Selector6/1 -> XudX2/1
  Selector5/1 -> XudX1/2
  Selector4/1 -> XudX1/1
  dXeff/1 -> Selector4/1, Selector6/1, Selector8/1, Selector10/1, Selector2/1
  Mux/1 -> Out1/1
  XudX1/1 -> Gain4/1
  XudX2/1 -> Gain6/1
  XudX3/1 -> Gain5/1
  XudX4/1 -> Gain7/1
  Selector2/1 -> XudXB/1

== system ctrl_PF_ad/HDM/HDM B3/Y/YdXi ==
  dX : Inport
  z : Inport  Port=2
  Mux : Mux
  Selector1 : Selector  InputPortWidth=5  IndexOptions=Index vector (dialog)  Indices=2  OutputSizes=1
  Selector2 : Selector  InputPortWidth=5  IndexOptions=Index vector (dialog)  Indices=3  OutputSizes=1
  Selector3 : Selector  InputPortWidth=5  IndexOptions=Index vector (dialog)  Indices=4  OutputSizes=1
  Selector7 : Selector  InputPortWidth=5  IndexOptions=Index vector (dialog)  Indices=1  OutputSizes=1
  YdX1 : Lookup_n-D  BreakpointsForDimension1=[-10 0 10]  BreakpointsForDimension2=|  BreakpointsForDimension3=[-5.14444 -3.08666664 -1.54332]  Table=|  InternalRulePriority=Speed  RndMeth=Simplest
      BreakpointsForDimension2=|
      | [-36.4062987
      | -18.4062987
      | -15.4062987
      | -13.9062987]
      Table=|
      | reshape([-1.8282E-04
      | -6.0037E-06
      | 1.6496E-04
      | -1.7978E-04
      | -2.4314E-06
      | 1.6969E-04
      | -1.4480E-04
      | -2.4314E-06
      | 2.0267E-04
      | -1.7641E-04
      | 1.4850E-06
      | 1.7514E-04],[3,4])
      settings: InputPortMap=u0,u1
  YdX2 : Lookup_n-D  BreakpointsForDimension1=[-10 0 10]  BreakpointsForDimension2=|  BreakpointsForDimension3=[-5.14444 -3.08666664 -1.54332]  Table=|  InternalRulePriority=Speed  RndMeth=Simplest
      BreakpointsForDimension2=|
      | [-36.4062987
      | -18.4062987
      | -15.4062987
      | -13.9062987]
      Table=|
      | reshape([1.4857E-04
      | -6.6611E-06
      | -1.5932E-04
      | 1.4200E-04
      | -1.2968E-05
      | -1.6860E-04
      | 9.4982E-05
      | -1.2968E-05
      | -2.1344E-04
      | 1.3366E-04
      | -2.3176E-05
      | -1.8599E-04],[3,4])
      settings: InputPortMap=u0,u1
  YdX3 : Lookup_n-D  BreakpointsForDimension1=[-10 0 10]  BreakpointsForDimension2=|  BreakpointsForDimension3=[-5.14444 -3.08666664 -1.54332]  Table=|  InternalRulePriority=Speed  RndMeth=Simplest
      BreakpointsForDimension2=|
      | [-36.4062987
      | -18.4062987
      | -15.4062987
      | -13.9062987]
      Table=|
      | reshape([2.0207E-04
      | 6.9701E-06
      | -1.9141E-04
      | 2.0588E-04
      | 1.3213E-05
      | -1.8007E-04
      | 2.2753E-04
      | 1.3213E-05
      | -1.0937E-04
      | 2.1222E-04
      | 2.3270E-05
      | -1.6161E-04],[3,4])
      settings: InputPortMap=u0,u1
  YdX4 : Lookup_n-D  BreakpointsForDimension1=[-10 0 10]  BreakpointsForDimension2=|  BreakpointsForDimension3=[-5.14444 -3.08666664 -1.54332]  Table=|  InternalRulePriority=Speed  RndMeth=Simplest
      BreakpointsForDimension2=|
      | [-36.4062987
      | -18.4062987
      | -15.4062987
      | -13.9062987]
      Table=|
      | reshape([-1.7022E-04
      | 5.9932E-06
      | 1.8722E-04
      | -1.7390E-04
      | 2.3770E-06
      | 1.8293E-04
      | -2.0489E-04
      | 2.3770E-06
      | 1.4658E-04
      | -1.7771E-04
      | -1.6689E-06
      | 1.7805E-04],[3,4])
      settings: InputPortMap=u0,u1
  YdX : Outport
  wires:
  Selector1/1 -> YdX2/1
  Selector2/1 -> YdX3/1
  Selector3/1 -> YdX4/1
  dX/1 -> Selector7/1, Selector1/1, Selector3/1, Selector2/1
  Selector7/1 -> YdX1/1
  YdX4/1 -> Mux/4
  YdX3/1 -> Mux/3
  YdX2/1 -> Mux/2
  YdX1/1 -> Mux/1
  z/1 -> YdX1/2, YdX2/2, YdX3/2, YdX4/2
  Mux/1 -> YdX/1
